simulink model "FSE"  (R2024a)
settings: Solver=ode45  StartTime=0.0  StopTime=2e3  RelTol=1e-3  EnableMultiTasking=on
PreLoadFcn:
  | FSE_PreLoadFcn
undefined symbols (not defined in the file): j, QAM, S, vsva2197, xcvc1902
libraries: hdlBasic x137, dspmlti4 x2, hdlUtilities x1, vmcUtilities x1
(part 2 of 2)

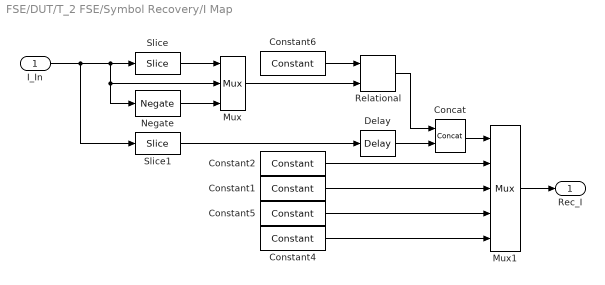
== system FSE/DUT/T_2 FSE/Symbol Recovery/I Map ==
  I_In : Inport
  Concat : hdlBasic/Concat  num_inputs=2  XmcBlockStatus=1  maskContainerNames=group1  block_type=concat  block_config=sysgen:Concat_config
  Constant1 : hdlBasic/Constant  const=-1/3  gui_display_data_type=Fixed-point  arith_type=Signed (2's comp)  n_bits=9  bin_pt=8  preci_type=Single  exp_width=8  frac_width=24  explicit_period=off  period=1  XmcBlockStatus=1  maskContainerNames=tabcontainer1  block_type=constant  block_config=sysgen:Constant_config
  Constant2 : hdlBasic/Constant  const=1/3  gui_display_data_type=Fixed-point  arith_type=Signed (2's comp)  n_bits=9  bin_pt=8  preci_type=Single  exp_width=8  frac_width=24  explicit_period=off  period=1  XmcBlockStatus=1  maskContainerNames=tabcontainer1  block_type=constant  block_config=sysgen:Constant_config
  Constant4 : hdlBasic/Constant  const=-1  gui_display_data_type=Fixed-point  arith_type=Signed (2's comp)  n_bits=2  bin_pt=0  preci_type=Single  exp_width=8  frac_width=24  explicit_period=off  period=1  XmcBlockStatus=1  maskContainerNames=tabcontainer1  block_type=constant  block_config=sysgen:Constant_config
  Constant5 : hdlBasic/Constant  const=1  gui_display_data_type=Fixed-point  arith_type=Signed (2's comp)  n_bits=2  bin_pt=0  preci_type=Single  exp_width=8  frac_width=24  explicit_period=off  period=1  XmcBlockStatus=1  maskContainerNames=tabcontainer1  block_type=constant  block_config=sysgen:Constant_config
  Constant6 : hdlBasic/Constant  const=2/3  gui_display_data_type=Fixed-point  arith_type=Unsigned  n_bits=8  bin_pt=8  preci_type=Single  exp_width=8  frac_width=24  explicit_period=off  period=1  XmcBlockStatus=1  maskContainerNames=tabcontainer1  block_type=constant  block_config=sysgen:Constant_config
  Delay : hdlBasic/Delay  rst=off  en=off  latency=1  reg_retiming=off  XmcBlockStatus=1  maskContainerNames=group1  block_type=delay  block_config=sysgen:Delay_config
  Mux : hdlBasic/Mux  inputs=2  en=off  latency=1  precision=Full  arith_type="Signed  (2's comp)"  n_bits=8  bin_pt=2  quantization=Truncate  overflow=Wrap  XmcBlockStatus=1  maskContainerNames=tabcontainer1  block_type=mux  block_config=sysgen:Mux_config
  Mux1 : hdlBasic/Mux  inputs=4  en=off  latency=1  precision=User Defined  arith_type="Signed  (2's comp)"  n_bits=10  bin_pt=8  quantization=Truncate  overflow=Wrap  XmcBlockStatus=1  maskContainerNames=tabcontainer1  block_type=mux  block_config=sysgen:Mux_config
  Negate : hdlBasic/Negate  precision=Full  arith_type=Unsigned  n_bits=18  bin_pt=10  quantization=Truncate  overflow=Wrap  en=off  latency=0  XmcBlockStatus=1  maskContainerNames=tabcontainer1  block_type=negate  block_config=sysgen:Negate_config
  Relational : hdlBasic/Relational  mode=a<b  op_type=Bool  en=off  latency=0  XmcBlockStatus=1  maskContainerNames=tabcontainer1  block_type=relational  block_config=sysgen:Relational_config
  Slice : hdlBasic/Slice  nbits=1  boolean_output=off  mode=Upper Bit Location + Width  bit1=0  base1=MSB of Input  bit0=0  base0=LSB of Input  XmcBlockStatus=1  maskContainerNames=group1  block_type=slice  block_config=sysgen:Slice_config
  Slice1 : hdlBasic/Slice  nbits=1  boolean_output=off  mode=Upper Bit Location + Width  bit1=0  base1=MSB of Input  bit0=0  base0=LSB of Input  XmcBlockStatus=1  maskContainerNames=group1  block_type=slice  block_config=sysgen:Slice_config
  Rec_I : Outport  VectorParamsAs1DForOutWhenUnconnected=off
  wires:
  Mux1/1 -> Rec_I/1
  Concat/1 -> Mux1/1
  Constant5/1 -> Mux1/4
  Constant4/1 -> Mux1/5
  Constant1/1 -> Mux1/3
  Constant2/1 -> Mux1/2
  Slice/1 -> Mux/1
  I_In/1 -> Slice/1, Negate/1, Mux/2, Slice1/1
  Negate/1 -> Mux/3
  Mux/1 -> Relational/2
  Constant6/1 -> Relational/1
  Relational/1 -> Concat/1
  Slice1/1 -> Delay/1
  Delay/1 -> Concat/2

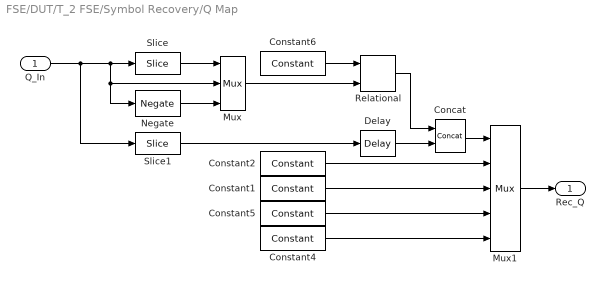
== system FSE/DUT/T_2 FSE/Symbol Recovery/Q Map ==
  Q_In : Inport
  Concat : hdlBasic/Concat  num_inputs=2  XmcBlockStatus=1  maskContainerNames=group1  block_type=concat  block_config=sysgen:Concat_config
  Constant1 : hdlBasic/Constant  const=-1/3  gui_display_data_type=Fixed-point  arith_type=Signed (2's comp)  n_bits=9  bin_pt=8  preci_type=Single  exp_width=8  frac_width=24  explicit_period=off  period=1  XmcBlockStatus=1  maskContainerNames=tabcontainer1  block_type=constant  block_config=sysgen:Constant_config
  Constant2 : hdlBasic/Constant  const=1/3  gui_display_data_type=Fixed-point  arith_type=Signed (2's comp)  n_bits=9  bin_pt=8  preci_type=Single  exp_width=8  frac_width=24  explicit_period=off  period=1  XmcBlockStatus=1  maskContainerNames=tabcontainer1  block_type=constant  block_config=sysgen:Constant_config
  Constant4 : hdlBasic/Constant  const=-1  gui_display_data_type=Fixed-point  arith_type=Signed (2's comp)  n_bits=2  bin_pt=0  preci_type=Single  exp_width=8  frac_width=24  explicit_period=off  period=1  XmcBlockStatus=1  maskContainerNames=tabcontainer1  block_type=constant  block_config=sysgen:Constant_config
  Constant5 : hdlBasic/Constant  const=1  gui_display_data_type=Fixed-point  arith_type=Signed (2's comp)  n_bits=2  bin_pt=0  preci_type=Single  exp_width=8  frac_width=24  explicit_period=off  period=1  XmcBlockStatus=1  maskContainerNames=tabcontainer1  block_type=constant  block_config=sysgen:Constant_config
  Constant6 : hdlBasic/Constant  const=2/3  gui_display_data_type=Fixed-point  arith_type=Unsigned  n_bits=8  bin_pt=8  preci_type=Single  exp_width=8  frac_width=24  explicit_period=off  period=1  XmcBlockStatus=1  maskContainerNames=tabcontainer1  block_type=constant  block_config=sysgen:Constant_config
  Delay : hdlBasic/Delay  rst=off  en=off  latency=1  reg_retiming=off  XmcBlockStatus=1  maskContainerNames=group1  block_type=delay  block_config=sysgen:Delay_config
  Mux : hdlBasic/Mux  inputs=2  en=off  latency=1  precision=Full  arith_type="Signed  (2's comp)"  n_bits=8  bin_pt=2  quantization=Truncate  overflow=Wrap  XmcBlockStatus=1  maskContainerNames=tabcontainer1  block_type=mux  block_config=sysgen:Mux_config
  Mux1 : hdlBasic/Mux  inputs=4  en=off  latency=1  precision=User Defined  arith_type="Signed  (2's comp)"  n_bits=10  bin_pt=8  quantization=Truncate  overflow=Wrap  XmcBlockStatus=1  maskContainerNames=tabcontainer1  block_type=mux  block_config=sysgen:Mux_config
  Negate : hdlBasic/Negate  precision=Full  arith_type=Unsigned  n_bits=18  bin_pt=10  quantization=Truncate  overflow=Wrap  en=off  latency=0  XmcBlockStatus=1  maskContainerNames=tabcontainer1  block_type=negate  block_config=sysgen:Negate_config
  Relational : hdlBasic/Relational  mode=a<b  op_type=Bool  en=off  latency=0  XmcBlockStatus=1  maskContainerNames=tabcontainer1  block_type=relational  block_config=sysgen:Relational_config
  Slice : hdlBasic/Slice  nbits=1  boolean_output=off  mode=Upper Bit Location + Width  bit1=0  base1=MSB of Input  bit0=0  base0=LSB of Input  XmcBlockStatus=1  maskContainerNames=group1  block_type=slice  block_config=sysgen:Slice_config
  Slice1 : hdlBasic/Slice  nbits=1  boolean_output=off  mode=Upper Bit Location + Width  bit1=0  base1=MSB of Input  bit0=0  base0=LSB of Input  XmcBlockStatus=1  maskContainerNames=group1  block_type=slice  block_config=sysgen:Slice_config
  Rec_Q : Outport  VectorParamsAs1DForOutWhenUnconnected=off
  wires:
  Mux1/1 -> Rec_Q/1
  Concat/1 -> Mux1/1
  Constant5/1 -> Mux1/4
  Constant4/1 -> Mux1/5
  Constant1/1 -> Mux1/3
  Constant2/1 -> Mux1/2
  Slice/1 -> Mux/1
  Q_In/1 -> Slice/1, Negate/1, Mux/2, Slice1/1
  Negate/1 -> Mux/3
  Mux/1 -> Relational/2
  Constant6/1 -> Relational/1
  Relational/1 -> Concat/1
  Slice1/1 -> Delay/1
  Delay/1 -> Concat/2

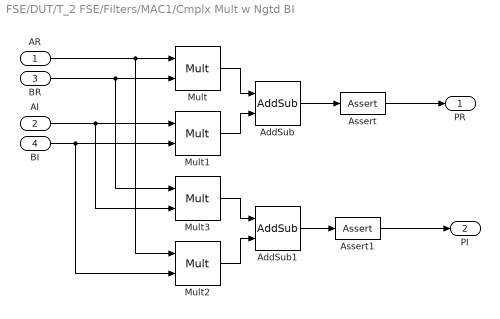
== system FSE/DUT/T_2 FSE/Filters/MAC1/Cmplx Mult w Ngtd BI ==
  AR : Inport
  AI : Inport  Port=2
  BR : Inport  Port=3
  BI : Inport  Port=4
  AddSub : hdlBasic/AddSub  mode=Addition  use_carryin=off  use_carryout=off  en=off  latency=1  precision=User Defined  arith_type="Signed  (2's comp)"  n_bits=36  bin_pt=28  quantization="Round  (unbiased: +/- Inf)"  overflow=Saturate  use_behavioral_HDL=on  hw_selection=Fabric  pipelined=off  use_rpm=off  XmcBlockStatus=1  maskContainerNames=tabcontainer1  block_type=addsub  block_config=sysgen:Addsub_config
  AddSub1 : hdlBasic/AddSub  mode=Subtraction  use_carryin=off  use_carryout=off  en=off  latency=1  precision=User Defined  arith_type="Signed  (2's comp)"  n_bits=36  bin_pt=28  quantization="Round  (unbiased: +/- Inf)"  overflow=Saturate  use_behavioral_HDL=on  hw_selection=Fabric  pipelined=off  use_rpm=off  XmcBlockStatus=1  maskContainerNames=tabcontainer1  block_type=addsub  block_config=sysgen:Addsub_config
  Assert : hdlBasic/Assert  assert_type=off  type_source=Explicitly  gui_display_data_type=Fixed-point  arith_type=Unsigned  n_bits=8  bin_pt=2  preci_type=Single  exp_width=8  frac_width=24  assert_rate=on  rate_source=Explicitly  period=1  output_port=on  XmcBlockStatus=1  maskContainerNames=group1  block_type=assert  block_config=sysgen:assert_config  block_width=609  block_height=900
  Assert1 : hdlBasic/Assert  assert_type=off  type_source=Explicitly  gui_display_data_type=Fixed-point  arith_type=Unsigned  n_bits=8  bin_pt=2  preci_type=Single  exp_width=8  frac_width=24  assert_rate=on  rate_source=Explicitly  period=1  output_port=on  XmcBlockStatus=1  maskContainerNames=group1  block_type=assert  block_config=sysgen:assert_config  block_width=609  block_height=900
  Mult : hdlBasic/Mult  precision=Full  arith_type="Signed  (2's comp)"  n_bits=36  bin_pt=28  quantization="Round  (unbiased: +/- Inf)"  overflow=Saturate  en=off  latency=2  opt_float=off  fp_mult_usage=No Usage  use_behavioral_HDL=off  opt=Speed  use_embedded=on  optimum_pipeline=off  pipeline=on  use_rpm=off  placement_style=Rectangular shape  XmcBlockStatus=1  maskContainerNames=group1  block_type=mult  block_config=sysgen:Mult_config  block_width=598  block_height=876
  Mult1 : hdlBasic/Mult  precision=Full  arith_type="Signed  (2's comp)"  n_bits=36  bin_pt=28  quantization="Round  (unbiased: +/- Inf)"  overflow=Saturate  en=off  latency=2  opt_float=off  fp_mult_usage=No Usage  use_behavioral_HDL=off  opt=Speed  use_embedded=on  optimum_pipeline=off  pipeline=on  use_rpm=off  placement_style=Rectangular shape  XmcBlockStatus=1  maskContainerNames=group1  block_type=mult  block_config=sysgen:Mult_config  block_width=598  block_height=876
  Mult2 : hdlBasic/Mult  precision=Full  arith_type="Signed  (2's comp)"  n_bits=36  bin_pt=28  quantization="Round  (unbiased: +/- Inf)"  overflow=Saturate  en=off  latency=2  opt_float=off  fp_mult_usage=No Usage  use_behavioral_HDL=off  opt=Speed  use_embedded=on  optimum_pipeline=off  pipeline=on  use_rpm=off  placement_style=Rectangular shape  XmcBlockStatus=1  maskContainerNames=group1  block_type=mult  block_config=sysgen:Mult_config  block_width=598  block_height=876
  Mult3 : hdlBasic/Mult  precision=Full  arith_type="Signed  (2's comp)"  n_bits=36  bin_pt=28  quantization=Truncate  overflow=Saturate  en=off  latency=2  opt_float=off  fp_mult_usage=No Usage  use_behavioral_HDL=off  opt=Speed  use_embedded=on  optimum_pipeline=off  pipeline=on  use_rpm=off  placement_style=Rectangular shape  XmcBlockStatus=1  maskContainerNames=group1  block_type=mult  block_config=sysgen:Mult_config  block_width=598  block_height=876
  PR : Outport  VectorParamsAs1DForOutWhenUnconnected=off
  PI : Outport  Port=2  VectorParamsAs1DForOutWhenUnconnected=off
  wires:
  AI/1 -> Mult3/2, Mult1/1
  BR/1 -> Mult3/1, Mult/2
  BI/1 -> Mult2/2, Mult1/2
  AR/1 -> Mult2/1, Mult/1
  Mult/1 -> AddSub/1
  Mult1/1 -> AddSub/2
  AddSub/1 -> Assert/1
  AddSub1/1 -> Assert1/1
  Mult3/1 -> AddSub1/1
  Mult2/1 -> AddSub1/2
  Assert/1 -> PR/1
  Assert1/1 -> PI/1

== system FSE/DUT/T_2 FSE/Filters/MAC1/Cmplx Mult1 ==
  AR : Inport
  AI : Inport  Port=2
  BR : Inport  Port=3
  BI : Inport  Port=4
  AddSub : hdlBasic/AddSub  mode=Subtraction  use_carryin=off  use_carryout=off  en=off  latency=2  precision=User Defined  arith_type="Signed  (2's comp)"  n_bits=36  bin_pt=28  quantization="Round  (unbiased: +/- Inf)"  overflow=Saturate  use_behavioral_HDL=on  hw_selection=Fabric  pipelined=off  use_rpm=off  XmcBlockStatus=1  maskContainerNames=tabcontainer1  block_type=addsub  block_config=sysgen:Addsub_config
  AddSub1 : hdlBasic/AddSub  mode=Addition  use_carryin=off  use_carryout=off  en=off  latency=2  precision=User Defined  arith_type="Signed  (2's comp)"  n_bits=36  bin_pt=28  quantization="Round  (unbiased: +/- Inf)"  overflow=Saturate  use_behavioral_HDL=on  hw_selection=Fabric  pipelined=off  use_rpm=off  XmcBlockStatus=1  maskContainerNames=tabcontainer1  block_type=addsub  block_config=sysgen:Addsub_config
  Mult : hdlBasic/Mult  precision=Full  arith_type="Signed  (2's comp)"  n_bits=36  bin_pt=28  quantization="Round  (unbiased: +/- Inf)"  overflow=Saturate  en=off  latency=2  opt_float=off  fp_mult_usage=No Usage  use_behavioral_HDL=off  opt=Speed  use_embedded=on  optimum_pipeline=off  pipeline=on  use_rpm=off  placement_style=Rectangular shape  XmcBlockStatus=1  maskContainerNames=group1  block_type=mult  block_config=sysgen:Mult_config  block_width=598  block_height=876
  Mult1 : hdlBasic/Mult  precision=Full  arith_type="Signed  (2's comp)"  n_bits=36  bin_pt=28  quantization="Round  (unbiased: +/- Inf)"  overflow=Saturate  en=off  latency=2  opt_float=off  fp_mult_usage=No Usage  use_behavioral_HDL=off  opt=Speed  use_embedded=on  optimum_pipeline=off  pipeline=on  use_rpm=off  placement_style=Rectangular shape  XmcBlockStatus=1  maskContainerNames=group1  block_type=mult  block_config=sysgen:Mult_config  block_width=598  block_height=876
  Mult2 : hdlBasic/Mult  precision=Full  arith_type="Signed  (2's comp)"  n_bits=36  bin_pt=28  quantization="Round  (unbiased: +/- Inf)"  overflow=Saturate  en=off  latency=2  opt_float=off  fp_mult_usage=No Usage  use_behavioral_HDL=off  opt=Speed  use_embedded=on  optimum_pipeline=off  pipeline=on  use_rpm=off  placement_style=Rectangular shape  XmcBlockStatus=1  maskContainerNames=group1  block_type=mult  block_config=sysgen:Mult_config  block_width=598  block_height=876
  Mult3 : hdlBasic/Mult  precision=Full  arith_type="Signed  (2's comp)"  n_bits=36  bin_pt=28  quantization=Truncate  overflow=Saturate  en=off  latency=2  opt_float=off  fp_mult_usage=No Usage  use_behavioral_HDL=off  opt=Speed  use_embedded=on  optimum_pipeline=off  pipeline=on  use_rpm=off  placement_style=Rectangular shape  XmcBlockStatus=1  maskContainerNames=group1  block_type=mult  block_config=sysgen:Mult_config  block_width=598  block_height=876
  PR : Outport  VectorParamsAs1DForOutWhenUnconnected=off
  PI : Outport  Port=2  VectorParamsAs1DForOutWhenUnconnected=off
  wires:
  AddSub1/1 -> PI/1
  AddSub/1 -> PR/1
  Mult3/1 -> AddSub1/2
  Mult2/1 -> AddSub1/1
  Mult1/1 -> AddSub/2
  Mult/1 -> AddSub/1
  AR/1 -> Mult2/1, Mult/1
  BI/1 -> Mult2/2, Mult1/2
  BR/1 -> Mult3/1, Mult/2
  AI/1 -> Mult3/2, Mult1/1

== system FSE/DUT/T_2 FSE/Filters/MAC1/Coeff Buffer ==
  In : Inport
  Addressable Shift Register : hdlBasic/Addressable Shift Register  infer_latency=on  depth=4  initVector=[0 0]  en=off  use_behavioral_HDL=off  Optimization=Resource  use_rpm=off  XmcBlockStatus=1  maskContainerNames=group1  block_type=addrsr  block_config=sysgen:Addrsr_config
  Constant : hdlBasic/Constant  const=1  gui_display_data_type=Fixed-point  arith_type=Unsigned  n_bits=1  bin_pt=0  preci_type=Single  exp_width=8  frac_width=24  explicit_period=on  period=1  XmcBlockStatus=1  maskContainerNames=tabcontainer1  block_type=constant  block_config=sysgen:Constant_config
  Register1 : hdlBasic/Register  init=0  rst=off  en=off  XmcBlockStatus=1  maskContainerNames=tabcontainer1  block_type=register  block_config=sysgen:Register_config
  Register6 : hdlBasic/Register  init=0  rst=off  en=off  XmcBlockStatus=1  maskContainerNames=tabcontainer1  block_type=register  block_config=sysgen:Register_config
  Out : Outport  VectorParamsAs1DForOutWhenUnconnected=off
  wires:
  Constant/1 -> Addressable Shift Register/2
  In/1 -> Register1/1
  Addressable Shift Register/1 -> Register6/1
  Register6/1 -> Out/1
  Register1/1 -> Addressable Shift Register/1

== system FSE/DUT/T_2 FSE/Filters/MAC1/Coeff Buffer1 ==
  In : Inport
  Addressable Shift Register : hdlBasic/Addressable Shift Register  infer_latency=on  depth=4  initVector=[0 0]  en=off  use_behavioral_HDL=off  Optimization=Resource  use_rpm=off  XmcBlockStatus=1  maskContainerNames=group1  block_type=addrsr  block_config=sysgen:Addrsr_config
  Constant : hdlBasic/Constant  const=1  gui_display_data_type=Fixed-point  arith_type=Unsigned  n_bits=1  bin_pt=0  preci_type=Single  exp_width=8  frac_width=24  explicit_period=on  period=1  XmcBlockStatus=1  maskContainerNames=tabcontainer1  block_type=constant  block_config=sysgen:Constant_config
  Register1 : hdlBasic/Register  init=0  rst=off  en=off  XmcBlockStatus=1  maskContainerNames=tabcontainer1  block_type=register  block_config=sysgen:Register_config
  Register6 : hdlBasic/Register  init=0  rst=off  en=off  XmcBlockStatus=1  maskContainerNames=tabcontainer1  block_type=register  block_config=sysgen:Register_config
  Out : Outport  VectorParamsAs1DForOutWhenUnconnected=off
  wires:
  Constant/1 -> Addressable Shift Register/2
  In/1 -> Register1/1
  Addressable Shift Register/1 -> Register6/1
  Register6/1 -> Out/1
  Register1/1 -> Addressable Shift Register/1

== system FSE/DUT/T_2 FSE/Filters/MAC2/Cmplx Mult w Ngtd BI ==
  AR : Inport
  AI : Inport  Port=2
  BR : Inport  Port=3
  BI : Inport  Port=4
  AddSub : hdlBasic/AddSub  mode=Addition  use_carryin=off  use_carryout=off  en=off  latency=1  precision=User Defined  arith_type="Signed  (2's comp)"  n_bits=36  bin_pt=28  quantization="Round  (unbiased: +/- Inf)"  overflow=Saturate  use_behavioral_HDL=on  hw_selection=Fabric  pipelined=off  use_rpm=off  XmcBlockStatus=1  maskContainerNames=tabcontainer1  block_type=addsub  block_config=sysgen:Addsub_config
  AddSub1 : hdlBasic/AddSub  mode=Subtraction  use_carryin=off  use_carryout=off  en=off  latency=1  precision=User Defined  arith_type="Signed  (2's comp)"  n_bits=36  bin_pt=28  quantization="Round  (unbiased: +/- Inf)"  overflow=Saturate  use_behavioral_HDL=on  hw_selection=Fabric  pipelined=off  use_rpm=off  XmcBlockStatus=1  maskContainerNames=tabcontainer1  block_type=addsub  block_config=sysgen:Addsub_config
  Mult : hdlBasic/Mult  precision=Full  arith_type="Signed  (2's comp)"  n_bits=36  bin_pt=28  quantization="Round  (unbiased: +/- Inf)"  overflow=Saturate  en=off  latency=2  opt_float=off  fp_mult_usage=No Usage  use_behavioral_HDL=off  opt=Speed  use_embedded=on  optimum_pipeline=off  pipeline=on  use_rpm=off  placement_style=Rectangular shape  XmcBlockStatus=1  maskContainerNames=group1  block_type=mult  block_config=sysgen:Mult_config  block_width=598  block_height=876
  Mult1 : hdlBasic/Mult  precision=Full  arith_type="Signed  (2's comp)"  n_bits=36  bin_pt=28  quantization="Round  (unbiased: +/- Inf)"  overflow=Saturate  en=off  latency=2  opt_float=off  fp_mult_usage=No Usage  use_behavioral_HDL=off  opt=Speed  use_embedded=on  optimum_pipeline=off  pipeline=on  use_rpm=off  placement_style=Rectangular shape  XmcBlockStatus=1  maskContainerNames=group1  block_type=mult  block_config=sysgen:Mult_config  block_width=598  block_height=876
  Mult2 : hdlBasic/Mult  precision=Full  arith_type="Signed  (2's comp)"  n_bits=36  bin_pt=28  quantization="Round  (unbiased: +/- Inf)"  overflow=Saturate  en=off  latency=2  opt_float=off  fp_mult_usage=No Usage  use_behavioral_HDL=off  opt=Speed  use_embedded=on  optimum_pipeline=off  pipeline=on  use_rpm=off  placement_style=Rectangular shape  XmcBlockStatus=1  maskContainerNames=group1  block_type=mult  block_config=sysgen:Mult_config  block_width=598  block_height=876
  Mult3 : hdlBasic/Mult  precision=Full  arith_type="Signed  (2's comp)"  n_bits=36  bin_pt=28  quantization=Truncate  overflow=Saturate  en=off  latency=2  opt_float=off  fp_mult_usage=No Usage  use_behavioral_HDL=off  opt=Speed  use_embedded=on  optimum_pipeline=off  pipeline=on  use_rpm=off  placement_style=Rectangular shape  XmcBlockStatus=1  maskContainerNames=group1  block_type=mult  block_config=sysgen:Mult_config  block_width=598  block_height=876
  PR : Outport  VectorParamsAs1DForOutWhenUnconnected=off
  PI : Outport  Port=2  VectorParamsAs1DForOutWhenUnconnected=off
  wires:
  AddSub1/1 -> PI/1
  AddSub/1 -> PR/1
  Mult1/1 -> AddSub/2
  Mult/1 -> AddSub/1
  AR/1 -> Mult2/1, Mult/1
  BI/1 -> Mult2/2, Mult1/2
  BR/1 -> Mult3/1, Mult/2
  AI/1 -> Mult3/2, Mult1/1
  Mult3/1 -> AddSub1/1
  Mult2/1 -> AddSub1/2

== system FSE/DUT/T_2 FSE/Filters/MAC2/Cmplx Mult1 ==
  AR : Inport
  AI : Inport  Port=2
  BR : Inport  Port=3
  BI : Inport  Port=4
  AddSub : hdlBasic/AddSub  mode=Subtraction  use_carryin=off  use_carryout=off  en=off  latency=2  precision=User Defined  arith_type="Signed  (2's comp)"  n_bits=36  bin_pt=28  quantization="Round  (unbiased: +/- Inf)"  overflow=Saturate  use_behavioral_HDL=on  hw_selection=Fabric  pipelined=off  use_rpm=off  XmcBlockStatus=1  maskContainerNames=tabcontainer1  block_type=addsub  block_config=sysgen:Addsub_config
  AddSub1 : hdlBasic/AddSub  mode=Addition  use_carryin=off  use_carryout=off  en=off  latency=2  precision=User Defined  arith_type="Signed  (2's comp)"  n_bits=36  bin_pt=28  quantization="Round  (unbiased: +/- Inf)"  overflow=Saturate  use_behavioral_HDL=on  hw_selection=Fabric  pipelined=off  use_rpm=off  XmcBlockStatus=1  maskContainerNames=tabcontainer1  block_type=addsub  block_config=sysgen:Addsub_config
  Mult : hdlBasic/Mult  precision=Full  arith_type="Signed  (2's comp)"  n_bits=36  bin_pt=28  quantization="Round  (unbiased: +/- Inf)"  overflow=Saturate  en=off  latency=2  opt_float=off  fp_mult_usage=No Usage  use_behavioral_HDL=off  opt=Speed  use_embedded=on  optimum_pipeline=off  pipeline=on  use_rpm=off  placement_style=Rectangular shape  XmcBlockStatus=1  maskContainerNames=group1  block_type=mult  block_config=sysgen:Mult_config  block_width=598  block_height=876
  Mult1 : hdlBasic/Mult  precision=Full  arith_type="Signed  (2's comp)"  n_bits=36  bin_pt=28  quantization="Round  (unbiased: +/- Inf)"  overflow=Saturate  en=off  latency=2  opt_float=off  fp_mult_usage=No Usage  use_behavioral_HDL=off  opt=Speed  use_embedded=on  optimum_pipeline=off  pipeline=on  use_rpm=off  placement_style=Rectangular shape  XmcBlockStatus=1  maskContainerNames=group1  block_type=mult  block_config=sysgen:Mult_config  block_width=598  block_height=876
  Mult2 : hdlBasic/Mult  precision=Full  arith_type="Signed  (2's comp)"  n_bits=36  bin_pt=28  quantization="Round  (unbiased: +/- Inf)"  overflow=Saturate  en=off  latency=2  opt_float=off  fp_mult_usage=No Usage  use_behavioral_HDL=off  opt=Speed  use_embedded=on  optimum_pipeline=off  pipeline=on  use_rpm=off  placement_style=Rectangular shape  XmcBlockStatus=1  maskContainerNames=group1  block_type=mult  block_config=sysgen:Mult_config  block_width=598  block_height=876
  Mult3 : hdlBasic/Mult  precision=Full  arith_type="Signed  (2's comp)"  n_bits=36  bin_pt=28  quantization=Truncate  overflow=Saturate  en=off  latency=2  opt_float=off  fp_mult_usage=No Usage  use_behavioral_HDL=off  opt=Speed  use_embedded=on  optimum_pipeline=off  pipeline=on  use_rpm=off  placement_style=Rectangular shape  XmcBlockStatus=1  maskContainerNames=group1  block_type=mult  block_config=sysgen:Mult_config  block_width=598  block_height=876
  PR : Outport  VectorParamsAs1DForOutWhenUnconnected=off
  PI : Outport  Port=2  VectorParamsAs1DForOutWhenUnconnected=off
  wires:
  AI/1 -> Mult3/2, Mult1/1
  BR/1 -> Mult3/1, Mult/2
  BI/1 -> Mult2/2, Mult1/2
  AR/1 -> Mult2/1, Mult/1
  Mult/1 -> AddSub/1
  Mult1/1 -> AddSub/2
  Mult2/1 -> AddSub1/1
  Mult3/1 -> AddSub1/2
  AddSub/1 -> PR/1
  AddSub1/1 -> PI/1

== system FSE/DUT/T_2 FSE/Filters/MAC2/Coeff Buffer ==
  In : Inport
  Addressable Shift Register : hdlBasic/Addressable Shift Register  infer_latency=on  depth=4  initVector=[1 0]  en=off  use_behavioral_HDL=off  Optimization=Resource  use_rpm=off  XmcBlockStatus=1  maskContainerNames=group1  block_type=addrsr  block_config=sysgen:Addrsr_config
  Constant : hdlBasic/Constant  const=1  gui_display_data_type=Fixed-point  arith_type=Unsigned  n_bits=1  bin_pt=0  preci_type=Single  exp_width=8  frac_width=24  explicit_period=on  period=1  XmcBlockStatus=1  maskContainerNames=tabcontainer1  block_type=constant  block_config=sysgen:Constant_config
  Register1 : hdlBasic/Register  init=0  rst=off  en=off  XmcBlockStatus=1  maskContainerNames=tabcontainer1  block_type=register  block_config=sysgen:Register_config
  Register6 : hdlBasic/Register  init=0  rst=off  en=off  XmcBlockStatus=1  maskContainerNames=tabcontainer1  block_type=register  block_config=sysgen:Register_config
  Out : Outport  VectorParamsAs1DForOutWhenUnconnected=off
  wires:
  Register6/1 -> Out/1
  Constant/1 -> Addressable Shift Register/2
  In/1 -> Register1/1
  Addressable Shift Register/1 -> Register6/1
  Register1/1 -> Addressable Shift Register/1

== system FSE/DUT/T_2 FSE/Filters/MAC2/Coeff Buffer1 ==
  In : Inport
  Addressable Shift Register : hdlBasic/Addressable Shift Register  infer_latency=on  depth=4  initVector=[0 0 0]  en=off  use_behavioral_HDL=off  Optimization=Resource  use_rpm=off  XmcBlockStatus=1  maskContainerNames=group1  block_type=addrsr  block_config=sysgen:Addrsr_config
  Constant : hdlBasic/Constant  const=1  gui_display_data_type=Fixed-point  arith_type=Unsigned  n_bits=1  bin_pt=0  preci_type=Single  exp_width=8  frac_width=24  explicit_period=on  period=1  XmcBlockStatus=1  maskContainerNames=tabcontainer1  block_type=constant  block_config=sysgen:Constant_config
  Register1 : hdlBasic/Register  init=0  rst=off  en=off  XmcBlockStatus=1  maskContainerNames=tabcontainer1  block_type=register  block_config=sysgen:Register_config
  Register6 : hdlBasic/Register  init=0  rst=off  en=off  XmcBlockStatus=1  maskContainerNames=tabcontainer1  block_type=register  block_config=sysgen:Register_config
  Out : Outport  VectorParamsAs1DForOutWhenUnconnected=off
  wires:
  Constant/1 -> Addressable Shift Register/2
  In/1 -> Register1/1
  Addressable Shift Register/1 -> Register6/1
  Register6/1 -> Out/1
  Register1/1 -> Addressable Shift Register/1
